simulink model "ModelFridgeEvaporatorSoln"  (R2024a)
settings: Solver=VariableStepAuto  StartTime=0.0  StopTime=3600  RelTol=1e-3  AbsTol=1e-3
libraries: fl_lib x19, nesl_utility x7, SimscapeFluids_lib x3
CloseFcn:
  | try,close(h1_step1_EvaporatorHarness),end
  | clear h1_step1_EvaporatorHarness
  | try,close(h2_step1_EvaporatorHarness),end
  | clear h2_step1_EvaporatorHarness
  | try,close(h3_step1_EvaporatorHarness),end
  | clear h3_step1_EvaporatorHarness
  | try,close(h4_step1_EvaporatorHarness),end
  | clear h4_step1_EvaporatorHarness
  | 
  | 
  | clear simlog_step1_EvaporatorHarness
  | clear logsout_step1_EvaporatorHarness
settings Model: Creator=emcgarri  LastModifiedBy=esmithzb
settings SolverCC: AutoScaleAbsTol=off  AlgebraicLoopSolver=TrustRegion  MaxZcPerStep=1
settings DataIOCC: MaxDataPoints=10000  SignalLoggingName=logsout_EvaporatorHarness
settings OptimizationCC: ReuseModelBlockBuffer=off
settings DebuggingCC: UnconnectedInputMsg=warning  UnconnectedOutputMsg=warning  UnconnectedLineMsg=warning  SymbolicDimsDataTypeCodeGenerationDiagnostic=none
settings ModelReferenceCC: EnableRefExpFcnMdlSchedulingChecks=on
settings SFSimCC: CustomCodeUndefinedFunction=UseInterfaceOnly
settings RTWCC: GPUComputeCapability=3.5  DLArmComputeVersion=19.05
settings SimscapeCC: SimscapeLogType=all  SimscapeLogSimulationStatistics=on  SimscapeLogName=simlog_EvaporatorHarness  SimscapeLogDataHistory=10000

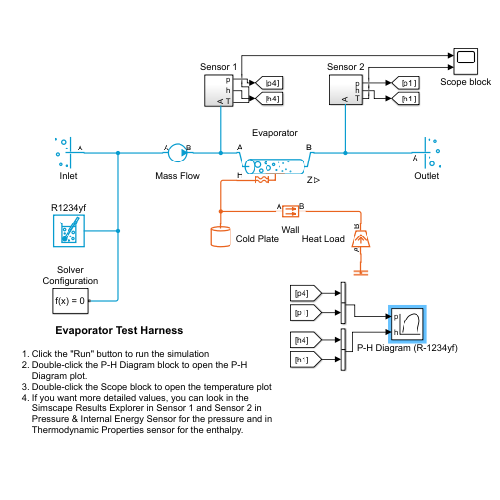
[thumbnail: Simulink's stored preview of the top-level diagram]
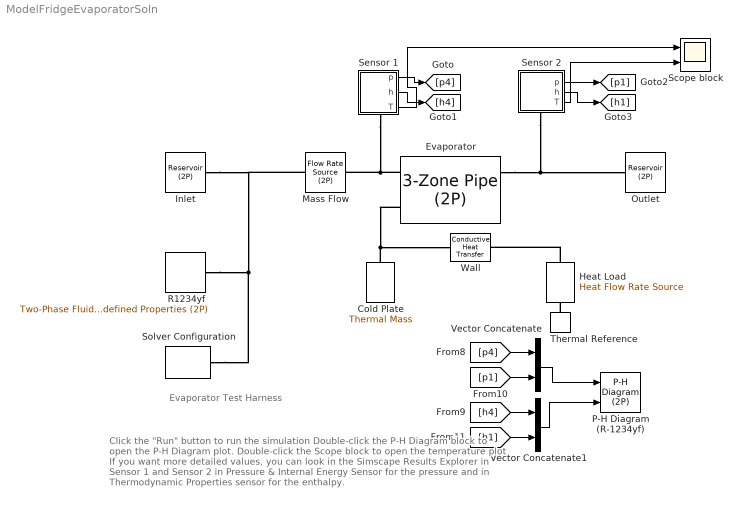
== system ModelFridgeEvaporatorSoln ==
  note: Click the "Run" button to run the simulation
      | Double-click the P-H Diagram block to open the P-H Diagram plot.
      | Double-click the Scope block to open the temperature plot
      | If you want more detailed values, you can look in the Simscape Results Explorer in Sensor 1 and Sensor 2 in Pressure & Internal Energy Sensor for the pressure and in Thermodynamic Properties sensor for the enthalpy.
  note: Evaporator Test Harness
  Cold Plate : fl_lib/Thermal/Thermal Elements/Thermal Mass  mass_type=foundation.enum.constant_variable.constant  mass=m_plate kg  sp_heat=cp_plate J/(K*kg)  mass_min=1e-6 kg  num_ports=foundation.enum.numPorts2.one  m_specify=off  m_priority=High  m=1 kg  m_nominal_specify=off  m_nominal_value=1  m_nominal_unit=kg  T_specify=on  T_priority=High  T=300 K  T_nominal_specify=off  T_nominal_value=1  T_nominal_unit=K  Q_specify=off  Q_priority=None  Q=0 W  Q_nominal_specify=off  Q_nominal_value=1  Q_nominal_unit=W
  Evaporator : SimscapeFluids_lib/Two-Phase Fluid/Pipes & Fittings/3-Zone Pipe (2P)  length=l_evap m  area=a_evap cm^2  Dh=d_evap cm  elevation_gain=0 m  g=9.81 m/s^2  length_add=0 m  roughness=15e-6 m  Re_lam=2000  Re_tur=4000  shape_factor=64  hc_ext=inf W/(m^2*K)  wall_thickness=t_wall mm  k_wall=k_plate W/(m*K)  c_wall=cp_plate J/(K*kg)  rho_wall=rho_plate kg/m^3  fin_ratio_ext=0  eta_fin_ext=0.5  fin_ratio_int=0  eta_fin_int=0.5  heat_coeff_spec=fluids.two_phase_fluid.pipes_fittings.enum.HeatCoeffSpec.GnielinskiCavalliniZecchin  colburn_coeff_liq=[.023, .8, .33]  colburn_coeff_mix=[.05, .8, .33]  colburn_coeff_vap=[.023, .8, .33]  Nu_lam=3.66  energy_spec=foundation.enum.energy_spec.enthalpy  p_init=p0_evap kPa  T_init=293.15 K  x_init=x0  alpha_init=0.5  h_init=h0_evap kJ/kg  u_init=1500 kJ/kg
      settings: InternalSimscapePortConfiguration="{\"Bottom\":[],\"Left\":[{\"id\":\"A\",\"label\":\"A\",\"type\":\"foundation.two_phase_fluid.two_phase_fluid\"},{\"id\":\"H\",\"label\":\"H\",\"type\":\"foundation.thermal.thermal\"}],\"Right\":[{\"id\":\"B\",\"label\":\"B\",\"type\":\"foundation.two_phase_fluid.two_phase_fluid\"},{\"id\":\"Z\",\"label\":\"Z\",\"type\":\"output\"}],\"Top\":[]}"
  Heat Load : fl_lib/Thermal/Thermal Sources/Heat Flow Rate Source  heat_flow=heat_load kW
      settings: InternalSimscapePortConfiguration="{\"Bottom\":[],\"Left\":[{\"id\":\"B\",\"label\":\"B\",\"type\":\"foundation.thermal.thermal\"}],\"Right\":[{\"id\":\"A\",\"label\":\"A\",\"type\":\"foundation.thermal.thermal\"}],\"Top\":[]}"
  Inlet : fl_lib/Two-Phase Fluid/Elements/Reservoir (2P)  pressure_spec=foundation.enum.ReservoirPressureSpec2P.Specified  reservoir_pressure=p0_evap kPa  reservoir_condensing_temperature=373.15 K  reservoir_evaporating_temperature=T0 K  energy_spec=foundation.enum.ReservoirEnergySpec2P.Enthalpy  reservoir_temperature=293.15 K  reservoir_quality=0.5  reservoir_void_fraction=0.5  reservoir_enthalpy=h0_evap kJ/kg  reservoir_internal_energy=1500 kJ/kg  reservoir_subcooling=5 deltaK  reservoir_superheating=5 deltaK  area_A=a_evap cm^2
  Mass Flow : fl_lib/Two-Phase Fluid/Sources/Flow Rate Source (2P)  source_type=foundation.enum.constant_controlled.constant  flow_type=foundation.enum.mass_volumetric_flow.mass  mass_flow=mdot_evap kg/s  volumetric_flow=0 m^3/s  power_spec=foundation.enum.power_spec.none  area_A=a_evap cm^2  area_B=a_evap cm^2
      settings: InternalSimscapePortConfiguration="{\"Bottom\":[],\"Left\":[{\"id\":\"A\",\"label\":\"A\",\"type\":\"foundation.two_phase_fluid.two_phase_fluid\"}],\"Right\":[{\"id\":\"B\",\"label\":\"B\",\"type\":\"foundation.two_phase_fluid.two_phase_fluid\"}],\"Top\":[]}"
  Outlet : fl_lib/Two-Phase Fluid/Elements/Reservoir (2P)  pressure_spec=foundation.enum.ReservoirPressureSpec2P.Specified  reservoir_pressure=p0_evap kPa  reservoir_condensing_temperature=373.15 K  reservoir_evaporating_temperature=T0 K  energy_spec=foundation.enum.ReservoirEnergySpec2P.Enthalpy  reservoir_temperature=293.15 K  reservoir_quality=0.5  reservoir_void_fraction=0.5  reservoir_enthalpy=h0_evap kJ/kg  reservoir_internal_energy=1500 kJ/kg  reservoir_subcooling=5 deltaK  reservoir_superheating=5 deltaK  area_A=a_evap cm^2
  P-H Diagram (R-1234yf) : SimscapeFluids_lib/Two-Phase Fluid/Utilities/P-H Diagram (2P)
  R1234yf : SimscapeFluids_lib/Two-Phase Fluid/Utilities/Two-Phase Fluid Predefined Properties (2P)  fluid=fluids.two_phase_fluid.utilities.enum.Fluid.R1234yf  p_atm=0.101325 MPa  properties_range_check=simscape.enum.assert.action.error  q_rev=0.01 Pa
  Scope block : Scope  NumInputPorts=2
  Sensor 1 : Subsystem
      settings: PortSchema="{\"entries\":[{\"content\":{\"sides\":[{\"content\":{\"connectorIds\":[]},\"type\":\"ConnectorPlacement.EquallySpacedRectSide\",\"uuid\":\"a2386ea4-012f-4d06-9e16-de8034e56d49\"},{\"content\":{\"connectorIds\":[\"Out1\",\"Out2\",\"Out3\"],\"side\":\"RIGHT\"},\"type\":\"ConnectorPlacement.EquallySpacedRectSide\",\"uuid\":\"4fc9eed4-9b91-4b18-836c-5d3d8d2a2391\"},{\"content\":{\"connectorIds\":[],\"side\":\"TOP\"},\"type\":\"ConnectorPlacement.EquallySpacedRectSide\",\"uuid\":\"63029c34-9cdb-4cf2-9461-f217553f00ec\"},{\"content\":{\"connectorIds\":[\"RConn1\"],\"side\":\"BOTTOM\"},\"type\":\"ConnectorPlacement.EquallySpacedRectSide\",\"uuid\":\"d2d8df23-35c6-4520-b0d8-5e88f3a56513\"}]},\"type\":\"ConnectorPlacement.EquallySpacedConnector\",\"uuid\":\"7866b668-ed43-4d72-8909-92d3adf450d4\"}],\"packageUris\":[\"http://schema.mathworks.com/mf0/Connector/R2020b\"],\"version\":\"1.0\"}"
  Sensor 2 : Subsystem
      settings: PortSchema="{\"entries\":[{\"content\":{\"sides\":[{\"content\":{\"connectorIds\":[]},\"type\":\"ConnectorPlacement.EquallySpacedRectSide\",\"uuid\":\"09a2fde7-9514-415f-ad1a-2358fbc90122\"},{\"content\":{\"connectorIds\":[\"Out1\",\"Out2\",\"Out3\"],\"side\":\"RIGHT\"},\"type\":\"ConnectorPlacement.EquallySpacedRectSide\",\"uuid\":\"1a58e595-65c2-481f-a4c6-044a1080df7a\"},{\"content\":{\"connectorIds\":[],\"side\":\"TOP\"},\"type\":\"ConnectorPlacement.EquallySpacedRectSide\",\"uuid\":\"e920d07f-3316-48c2-b5dc-69759bfb2eca\"},{\"content\":{\"connectorIds\":[\"RConn1\"],\"side\":\"BOTTOM\"},\"type\":\"ConnectorPlacement.EquallySpacedRectSide\",\"uuid\":\"ceb1a63b-e9f5-46e4-b72f-4e0e29463411\"}]},\"type\":\"ConnectorPlacement.EquallySpacedConnector\",\"uuid\":\"10759918-f7d5-4efa-b411-b89b519c736f\"}],\"packageUris\":[\"http://schema.mathworks.com/mf0/Connector/R2020b\"],\"version\":\"1.0\"}"
  Solver Configuration : nesl_utility/Solver Configuration  PhysicalDomain=network_engine_domain  SubClassName=solver  LeftPortType=input  RightPortType=generic  Tones=[]  Harmonics=[]  SimulateNoise=off  Profile=off  UseLocalSampling=off  EnableSwitchedLinearOptims=on  FrequencyDomain=off  UseCCode=off  RelTol=0.001  AbsTol=1e-06  MinStep=1e-09  ToWorkspace=off  RevertToSquareIcSolve=off  NumHomotopyIterations=100  PhasorMode=off  PhasorModeNumHarmonics=1  ConsistencySolver=NEWTON_XTOL_AFTER_FTOL  IndexReductionMethod=DerivativeReplacement  DoDC=on  ResidualTolerance=1e-09  ConsistencyTolSource=GLOBAL  ConsistencyAbsTol=0.001  ConsistencyRelTol=0.001  ConsistencyTolFactor=0.001  UseLocalSolver=off  LocalSolverChoice=NE_BACKWARD_EULER_ADVANCER  ResolveIndetEquations=on  FunctionEvalNumThread=1  LocalSolverSampleTime=0.001  DoFixedCost=off  MaxNonlinIter=3  MaxModeIter=2  ComputeImpulses=off  ImpulseIterations=2  LinearAlgebra=auto  LinearAlgebraNumThread=0  EquationFormulation=NE_TIME_EF  DelaysMemoryBudget=1024  AutomaticFiltering=on  FilteringTimeConstant=0.001  PartitionStorageMethod=AS_NEEDED  PartitionMemoryBudget=1024  PartitionMethod=ROBUST  MultibodyUseLocalSolver=off  MultibodyLocalSolverChoice=ODE1  MultibodyLocalSolverSampleTime=0.001
  Thermal Reference : fl_lib/Thermal/Thermal Elements/Thermal Reference
  Vector Concatenate : Concatenate
  Vector Concatenate1 : Concatenate
  Wall : fl_lib/Thermal/Thermal Elements/Conductive Heat Transfer  thermal_type=foundation.enum.ConstantVariableTabulated.Constant  wall_geometry=foundation.enum.ConductionWallGeometry.Planar  area=a_plate cm^2  thickness=t_cond_plate cm  d_in=0.05 m  d_out=0.1 m  L=1 m  th_cond_min=10 W/(K*m)  th_cond=k_plate W/(m*K)  th_cond_TLU=[413, 401, 392, 383, 371, 357, 342] W/(K*m)  temp_TLU=[200, 273, 400, 600, 800, 1000, 1200] K  T_specify=off  T_priority=None  T=0 K  T_nominal_specify=off  T_nominal_value=1  T_nominal_unit=K  Q_specify=off  Q_priority=None  Q=0 W  Q_nominal_specify=off  Q_nominal_value=1  Q_nominal_unit=W
  wires:
  Sensor 1/1(p) -> [p4]
  Sensor 1/2(h) -> [h4]
  Sensor 2/1(p) -> [p1]
  Sensor 2/2(h) -> [h1]
  [h4] -> Vector Concatenate1/1
  Vector Concatenate1/1 -> P-H Diagram (R-1234yf)/2
  Vector Concatenate/1 -> P-H Diagram (R-1234yf)/1
  [p1] -> Vector Concatenate/2
  [h1] -> Vector Concatenate1/2
  [p4] -> Vector Concatenate/1
  Sensor 1/3(T) -> Scope block/1
  Sensor 2/3(T) -> Scope block/2
  connections:
  Cold Plate/LConn1 -- Evaporator/LConn2 -- Wall/LConn1
  Heat Load/LConn1 -- Wall/RConn1
  Solver Configuration/RConn1 -- R1234yf/RConn1 -- Inlet/LConn1 -- Mass Flow/LConn1
  Thermal Reference/LConn1 -- Heat Load/RConn1
  Evaporator/RConn1 -- Outlet/LConn1 -- Sensor 2/RConn1
  Evaporator/LConn1 -- Sensor 1/RConn1 -- Mass Flow/RConn1

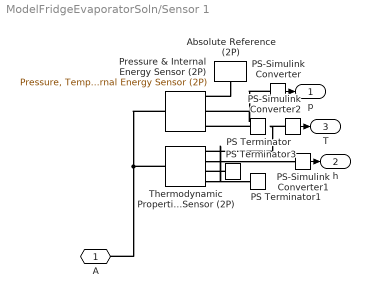
== system ModelFridgeEvaporatorSoln/Sensor 1 ==
  Absolute Reference (2P) : fl_lib/Two-Phase Fluid/Elements/Absolute Reference (2P)
  PS Terminator : fl_lib/Physical Signals/Sinks/PS Terminator
  PS Terminator1 : fl_lib/Physical Signals/Sinks/PS Terminator
  PS Terminator3 : fl_lib/Physical Signals/Sinks/PS Terminator
  PS-Simulink Converter : nesl_utility/PS-Simulink Converter  PhysicalDomain=network_engine_domain  SubClassName=ps_output  LeftPortType=input  RightPortType=output  PseudoPeriodic=off  Frequencies=[]  VectorFormat=1-D array  Unit=MPa  AffineConversion=off
  PS-Simulink Converter1 : nesl_utility/PS-Simulink Converter  PhysicalDomain=network_engine_domain  SubClassName=ps_output  LeftPortType=input  RightPortType=output  PseudoPeriodic=off  Frequencies=[]  VectorFormat=1-D array  Unit=kJ/kg  AffineConversion=off
  PS-Simulink Converter2 : nesl_utility/PS-Simulink Converter  PhysicalDomain=network_engine_domain  SubClassName=ps_output  LeftPortType=input  RightPortType=output  PseudoPeriodic=off  Frequencies=[]  VectorFormat=1-D array  Unit=K  AffineConversion=off
  Pressure & Internal Energy Sensor (2P) : fl_lib/Two-Phase Fluid/Sensors/Pressure, Temperature & Internal Energy Sensor (2P)  reference=foundation.enum.MeasurementReference.difference  pressure=true  pressure_spec=foundation.enum.PressureMeasementSpec.Absolute  temperature=false  internal_energy=true
      settings: InternalSimscapePortConfiguration="{\"Bottom\":[{\"id\":\"U\",\"label\":\"U\",\"type\":\"output\"}],\"Left\":[{\"id\":\"A\",\"label\":\"A\",\"type\":\"foundation.two_phase_fluid.two_phase_fluid\"}],\"Right\":[{\"id\":\"B\",\"label\":\"B\",\"type\":\"foundation.two_phase_fluid.two_phase_fluid\"},{\"id\":\"P\",\"label\":\"P\",\"type\":\"output\"}],\"Top\":[]}"
  Thermodynamic Properties Sensor (2P) : fl_lib/Two-Phase Fluid/Sensors/Thermodynamic Properties Sensor (2P)  temperature=true  enthalpy=true  density=false  specific_volume=true  entropy=true
      settings: InternalSimscapePortConfiguration="{\"Bottom\":[{\"id\":\"V\",\"label\":\"v\",\"type\":\"output\"},{\"id\":\"S\",\"label\":\"s\",\"type\":\"output\"}],\"Left\":[{\"id\":\"A\",\"label\":\"A\",\"type\":\"foundation.two_phase_fluid.two_phase_fluid\"}],\"Right\":[{\"id\":\"T\",\"label\":\"T\",\"type\":\"output\"},{\"id\":\"H\",\"label\":\"h\",\"type\":\"output\"}],\"Top\":[]}"
  A : PMIOPort  Side=Right
  p : Outport
  h : Outport  Port=2
  T : Outport  Port=3
  wires:
  PS-Simulink Converter/1 -> p/1
  PS-Simulink Converter1/1 -> h/1
  PS-Simulink Converter2/1 -> T/1
  connections:
  Thermodynamic Properties Sensor (2P)/RConn4 -- PS Terminator1/LConn1
  Absolute Reference (2P)/LConn1 -- Pressure & Internal Energy Sensor (2P)/RConn1
  Pressure & Internal Energy Sensor (2P)/LConn1 -- A/RConn1 -- Thermodynamic Properties Sensor (2P)/LConn1
  PS Terminator/LConn1 -- Pressure & Internal Energy Sensor (2P)/RConn3
  PS Terminator3/LConn1 -- Thermodynamic Properties Sensor (2P)/RConn3
  PS-Simulink Converter/LConn1 -- Pressure & Internal Energy Sensor (2P)/RConn2
  Thermodynamic Properties Sensor (2P)/RConn2 -- PS-Simulink Converter1/LConn1
  PS-Simulink Converter2/LConn1 -- Thermodynamic Properties Sensor (2P)/RConn1

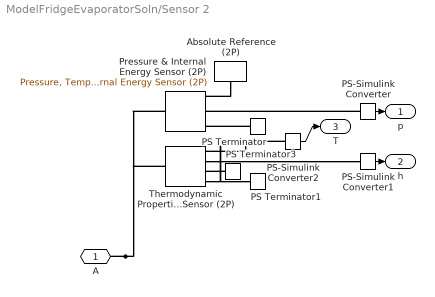
== system ModelFridgeEvaporatorSoln/Sensor 2 ==
  Absolute Reference (2P) : fl_lib/Two-Phase Fluid/Elements/Absolute Reference (2P)
  PS Terminator : fl_lib/Physical Signals/Sinks/PS Terminator
  PS Terminator1 : fl_lib/Physical Signals/Sinks/PS Terminator
  PS Terminator3 : fl_lib/Physical Signals/Sinks/PS Terminator
  PS-Simulink Converter : nesl_utility/PS-Simulink Converter  PhysicalDomain=network_engine_domain  SubClassName=ps_output  LeftPortType=input  RightPortType=output  PseudoPeriodic=off  Frequencies=[]  VectorFormat=1-D array  Unit=MPa  AffineConversion=off
  PS-Simulink Converter1 : nesl_utility/PS-Simulink Converter  PhysicalDomain=network_engine_domain  SubClassName=ps_output  LeftPortType=input  RightPortType=output  PseudoPeriodic=off  Frequencies=[]  VectorFormat=1-D array  Unit=kJ/kg  AffineConversion=off
  PS-Simulink Converter2 : nesl_utility/PS-Simulink Converter  PhysicalDomain=network_engine_domain  SubClassName=ps_output  LeftPortType=input  RightPortType=output  PseudoPeriodic=off  Frequencies=[]  VectorFormat=1-D array  Unit=K  AffineConversion=off
  Pressure & Internal Energy Sensor (2P) : fl_lib/Two-Phase Fluid/Sensors/Pressure, Temperature & Internal Energy Sensor (2P)  reference=foundation.enum.MeasurementReference.difference  pressure=true  pressure_spec=foundation.enum.PressureMeasementSpec.Absolute  temperature=false  internal_energy=true
      settings: InternalSimscapePortConfiguration="{\"Bottom\":[{\"id\":\"U\",\"label\":\"U\",\"type\":\"output\"}],\"Left\":[{\"id\":\"A\",\"label\":\"A\",\"type\":\"foundation.two_phase_fluid.two_phase_fluid\"}],\"Right\":[{\"id\":\"B\",\"label\":\"B\",\"type\":\"foundation.two_phase_fluid.two_phase_fluid\"},{\"id\":\"P\",\"label\":\"P\",\"type\":\"output\"}],\"Top\":[]}"
  Thermodynamic Properties Sensor (2P) : fl_lib/Two-Phase Fluid/Sensors/Thermodynamic Properties Sensor (2P)  temperature=true  enthalpy=true  density=false  specific_volume=true  entropy=true
      settings: InternalSimscapePortConfiguration="{\"Bottom\":[{\"id\":\"V\",\"label\":\"v\",\"type\":\"output\"},{\"id\":\"S\",\"label\":\"s\",\"type\":\"output\"}],\"Left\":[{\"id\":\"A\",\"label\":\"A\",\"type\":\"foundation.two_phase_fluid.two_phase_fluid\"}],\"Right\":[{\"id\":\"T\",\"label\":\"T\",\"type\":\"output\"},{\"id\":\"H\",\"label\":\"h\",\"type\":\"output\"}],\"Top\":[]}"
  A : PMIOPort  Side=Right
  p : Outport
  h : Outport  Port=2
  T : Outport  Port=3
  wires:
  PS-Simulink Converter1/1 -> h/1
  PS-Simulink Converter/1 -> p/1
  PS-Simulink Converter2/1 -> T/1
  connections:
  Thermodynamic Properties Sensor (2P)/RConn2 -- PS-Simulink Converter1/LConn1
  PS-Simulink Converter/LConn1 -- Pressure & Internal Energy Sensor (2P)/RConn2
  PS Terminator3/LConn1 -- Thermodynamic Properties Sensor (2P)/RConn3
  PS Terminator/LConn1 -- Pressure & Internal Energy Sensor (2P)/RConn3
  A/RConn1 -- Pressure & Internal Energy Sensor (2P)/LConn1 -- Thermodynamic Properties Sensor (2P)/LConn1
  Absolute Reference (2P)/LConn1 -- Pressure & Internal Energy Sensor (2P)/RConn1
  Thermodynamic Properties Sensor (2P)/RConn4 -- PS Terminator1/LConn1
  PS-Simulink Converter2/LConn1 -- Thermodynamic Properties Sensor (2P)/RConn1
